simulink model "RC"  (R2015a)
settings: Solver=ode45  StartTime=0.0  StopTime=20  RelTol=1e-3
libraries: powerlib x10
settings Model: Creator=maitr  LastModifiedBy=baoch

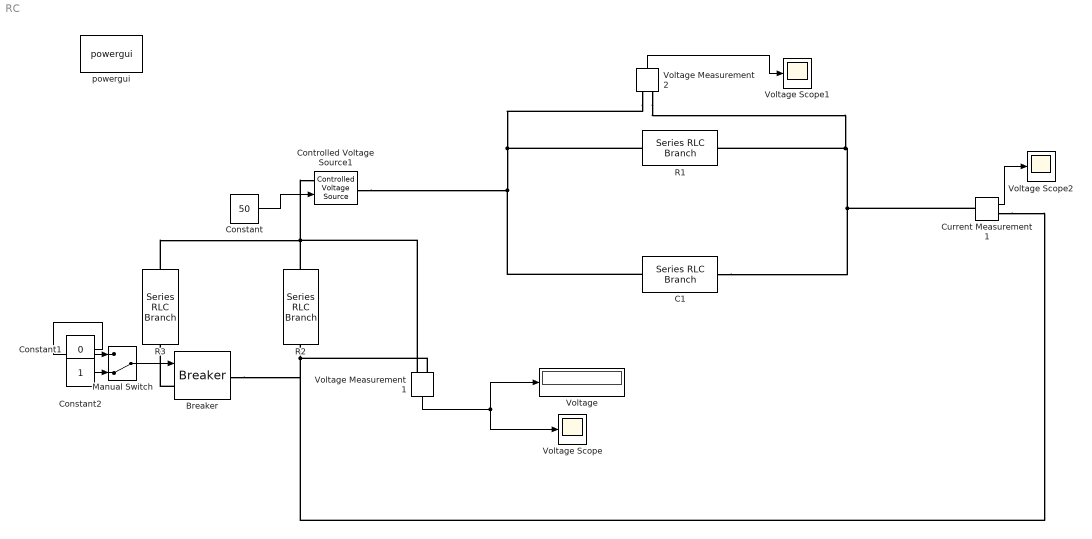
== system RC ==
  Breaker : powerlib/Elements/Breaker  InitialState=0  SwitchingTimes="[1/60  5/60]"  External=on  BreakerResistance=0.01  SnubberResistance=1e6  SnubberCapacitance=inf  Measurements=None  MoreParameters=on  NoBreakLoop=off
  C1 : powerlib/Elements/Series RLC Branch  LConnTagsString=__new0  RConnTagsString=__new0  BranchType=C  Resistance=1  Inductance=1e-3  SetiL0=off  InitialCurrent=0  Capacitance=1  Setx0=on  InitialVoltage=0  Measurements=None
  Constant : Constant  Value=50
  Constant1 : Constant  Value=0
  Constant2 : Constant
  Controlled Voltage Source1 : powerlib/Electrical Sources/Controlled Voltage Source  Initialize=on  Source_Type=DC  Amplitude=400  Phase=0  Frequency=0  Measurements=None
  Current Measurement1 : powerlib/Measurements/Current Measurement  PhasorSimulation=off  OutputType=Complex  PSBequivalent=0
  Manual Switch : ManualSwitch  CurrentSetting=0
  R1 : powerlib/Elements/Series RLC Branch  LConnTagsString=__new0  RConnTagsString=__new0  BranchType=R  Resistance=1  Inductance=1e-3  SetiL0=off  InitialCurrent=0  Capacitance=1e-6  Setx0=off  InitialVoltage=0  Measurements=None
  R2 : powerlib/Elements/Series RLC Branch  LConnTagsString=__new0  RConnTagsString=__new0  BranchType=R  Resistance=5  Inductance=1e-3  SetiL0=off  InitialCurrent=0  Capacitance=1e-6  Setx0=off  InitialVoltage=0  Measurements=None
  R3 : powerlib/Elements/Series RLC Branch  LConnTagsString=__new0  RConnTagsString=__new0  BranchType=R  Resistance=5  Inductance=1e-3  SetiL0=off  InitialCurrent=0  Capacitance=1e-6  Setx0=off  InitialVoltage=0  Measurements=None
  Voltage : Display
  Voltage Measurement1 : powerlib/Measurements/Voltage Measurement  PhasorSimulation=off  OutputType=Complex  PSBequivalent=0
  Voltage Measurement2 : powerlib/Measurements/Voltage Measurement  PhasorSimulation=off  OutputType=Complex  PSBequivalent=0
  Voltage Scope : Scope
      settings: TimeRange=20  YMin=25  YMax=50
  Voltage Scope1 : Scope
      settings: TimeRange=20  YMin=0  YMax=25
  Voltage Scope2 : Scope
      settings: TimeRange=20  YMin=8  YMax=17  SaveName=ScopeData2
  powergui : powerlib/powergui  Priority=1  SimulationMode=Discrete  SolverType=Tustin/Backward Euler (TBE)  SampleTime=0.000005  frequency=60  SPID=off  DisableSnubberDevices=off  DisableRonSwitches=off  DisableVfSwitches=off  SwTol=0  DisplayEquations=off  Interpol=off  methode=off  Ts=100  FunctionMessages=off  echomessages=off  HookPort=off  EnableUseOfTLC=off  x0status=blocks  frequencyindice=0  Pbase=100e6  ErrMax=1e-4  Iterations=50  UnitsV=kV  UnitsW=MW  buscounter=0  RestoreLinks=warning  ResistiveCurrentMeasurement=off  Frange=[0:2:500]  Ylog=off  Xlog=on  ShowGrid=off  save=off  variable=ZData  structure=0  ZoomFFT=off  StartTime=0.0  cycles=1  DisplayStyle=1  fundamental=60  FreqAxis=off  MaxFrequency=1000  frequencyindicesteady=1  RmsSteady=1  display=off
  wires:
  Voltage Measurement1/1 -> Voltage/1, Voltage Scope/1
  Current Measurement1/1 -> Voltage Scope2/1
  Constant/1 -> Controlled Voltage Source1/1
  Voltage Measurement2/1 -> Voltage Scope1/1
  Manual Switch/1 -> Breaker/1
  Constant2/1 -> Manual Switch/2
  Constant1/1 -> Manual Switch/1
  connections:
  R1/LConn1 -- Voltage Measurement2/LConn1 -- C1/LConn1 -- Controlled Voltage Source1/RConn1
  Current Measurement1/LConn1 -- C1/RConn1 -- Voltage Measurement2/LConn2 -- R1/RConn1
  R2/RConn1 -- R3/RConn1 -- Controlled Voltage Source1/LConn1 -- Voltage Measurement1/LConn2
  Current Measurement1/RConn1 -- Breaker/RConn1 -- Voltage Measurement1/LConn1 -- R2/LConn1
  Breaker/LConn1 -- R3/LConn1
